simulink model "GyroSimulationAndIdentification_2016a"  (R2016a)
settings: Solver=ode45  SolverMode=SingleTasking  StartTime=0.0  StopTime=70.0  RelTol=1e-3
InitFcn:
  | InitGyro
values from neighbouring files (symbols this model uses):
  alpha1 = history1.x((2*m*(iter1-1) + m + 1):(2*m*iter1))    [PlotDualVariables.m]
  alpha1_star = history1.x((2*m*(iter1-1) + 1):(2*m*(iter1-1) + m))    [PlotDualVariables.m]
  alpha2 = history2.x((2*m*(iter2-1) + m + 1):(2*m*iter2))    [PlotDualVariables.m]
  alpha2_star = history2.x((2*m*(iter2-1) + 1):(2*m*(iter2-1) + m))    [PlotDualVariables.m]
  alpha3 = history3.x((2*m*(iter3-1) + m + 1):(2*m*iter3))    [PlotDualVariables.m]
  alpha3_star = history3.x((2*m*(iter3-1) + 1):(2*m*(iter3-1) + m))    [PlotDualVariables.m]
  alpha4 = history4.x((2*m*(iter4-1) + m + 1):(2*m*iter4))    [PlotDualVariables.m]
  alpha4_star = history4.x((2*m*(iter4-1) + 1):(2*m*(iter4-1) + m))    [PlotDualVariables.m]
  alpha5 = history5.x((2*m*(iter5-1) + m + 1):(2*m*iter5))    [PlotDualVariables.m]
  alpha5_star = history5.x((2*m*(iter5-1) + 1):(2*m*(iter5-1) + m))    [PlotDualVariables.m]
  alpha6 = history6.x((2*m*(iter6-1) + m + 1):(2*m*iter6))    [PlotDualVariables.m]
  alpha6_star = history6.x((2*m*(iter6-1) + 1):(2*m*(iter6-1) + m))    [PlotDualVariables.m]
  alpha7 = history7.x((2*m*(iter7-1) + m + 1):(2*m*iter7))    [PlotDualVariables.m]
  alpha7_star = history7.x((2*m*(iter7-1) + 1):(2*m*(iter7-1) + m))    [PlotDualVariables.m]
  alpha8 = history8.x((2*m*(iter8-1) + m + 1):(2*m*iter8))    [PlotDualVariables.m]
  alpha8_star = history8.x((2*m*(iter8-1) + 1):(2*m*(iter8-1) + m))    [PlotDualVariables.m]
  I_test = (1/m)*ones(1,m)    [Main.m]
  Im = (1/m)*ones(m,m)    [Main.m]
  K = zeros(m,m)    [Main.m]
  K_test = zeros(1,m)    [Main.m]
  Kernel_Var = 0.01    [Main.m]
  m = 100    [Main.m]
  n = 10    [Main.m]
  q1dot_0 = 45    [RunMe.m]
  q2_0 = 0    [RunMe.m]
  q3_0 = 0    [RunMe.m]
  rhodata = rho_data.data(1:5000,:)    [Main.m]
  xopt = [ydata(1:m,:) udata(1:m,:)]    [Main.m]
undefined symbols (not defined in the file or in its folder): Dr, Du, sigbuilder_block
undefined symbols (not defined in the file): sys
libraries: simulink_extras x5, simulink x2, cstblocks x1
settings Model: Creator=jt  LastModifiedBy=Saeed
settings DataIOCC: LimitDataPoints=on  SaveFormat=Array
settings OptimizationCC: BlockReduction=off  BooleanDataType=off
settings DebuggingCC: SaveWithParameterizedLinksMsg=none  UnderspecifiedInitializationDetection=Classic  MergeDetectMultiDrivingBlocksExec=none  SignalResolutionControl=TryResolveAllWithWarning
settings HardwareCC: ProdBitPerPointer=32  ProdLargestAtomicFloat=None  ProdIntDivRoundTo=Undefined  ProdEndianess=Unspecified  ProdWordSize=32  ProdHWDeviceType=32-bit Generic  TargetUnknown=on
settings ModelReferenceCC: PropagateSignalLabelsOutOfModel=off
settings ConfigComp: CovSFcnEnable=off

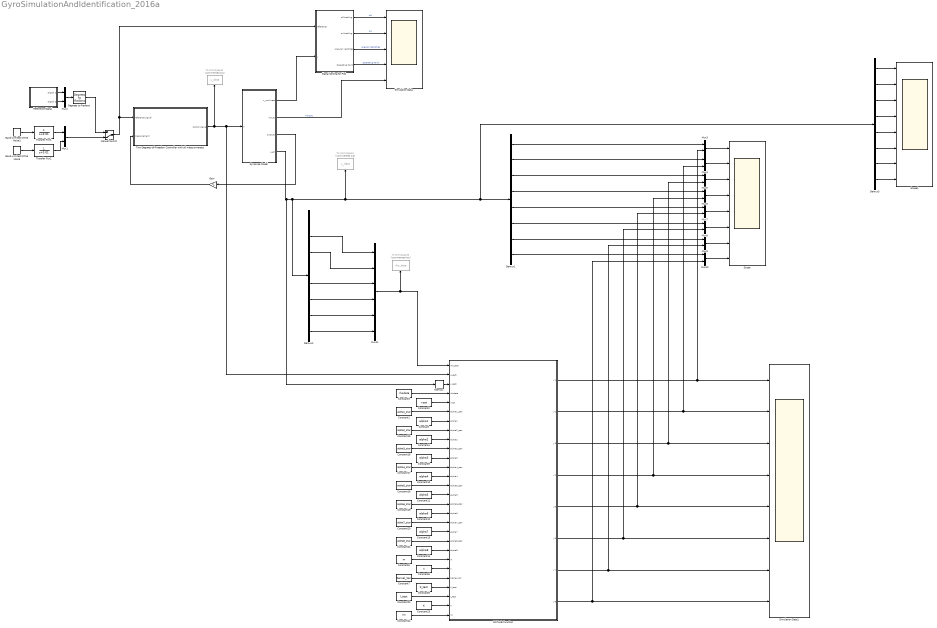
== system GyroSimulationAndIdentification_2016a ==
  Band-Limited White Noise : simulink/Sources/Band-Limited White Noise  Cov=[0.01]  Ts=0.01  seed=[3453]
  Band-Limited White Noise1 : simulink/Sources/Band-Limited White Noise  Cov=[0.01]  Ts=0.01  seed=[23341]
  Constant : Constant  Value=alpha1
  Constant1 : Constant  Value=alpha1_star
  Constant10 : Constant  Value=alpha4
  Constant11 : Constant  Value=alpha5
  Constant12 : Constant  Value=alpha6
  Constant13 : Constant  Value=alpha7
  Constant14 : Constant  Value=alpha8
  Constant15 : Constant  Value=alpha2_star
  Constant16 : Constant  Value=alpha3_star
  Constant17 : Constant  Value=alpha4_star
  Constant18 : Constant  Value=alpha5_star
  Constant19 : Constant  Value=alpha6_star
  Constant2 : Constant  Value=xopt
  Constant20 : Constant  Value=alpha7_star
  Constant21 : Constant  Value=alpha8_star
  Constant22 : Constant  Value=I_test
  Constant23 : Constant  Value=K
  Constant24 : Constant  Value=Im
  Constant3 : Constant  Value=rhodata
  Constant4 : Constant  Value=alpha2
  Constant5 : Constant  Value=m
  Constant6 : Constant  Value=n
  Constant7 : Constant  Value=Kernel_Var
  Constant8 : Constant  Value=K_test
  Constant9 : Constant  Value=alpha3
  Degrees to Radians : simulink_extras/Transformations/Degrees to Radians
  Demux1 : Demux  Outputs=8
  Demux2 : Demux  Outputs=8
  Demux3 : Demux  Outputs=8
  Gain : Gain  Gain=-1
  Gyroscpe Model : Subsystem
  MATLAB Function : MATLAB Function  TreatAsAtomicUnit=on
  Manual Switch : ManualSwitch  CurrentSetting=0
  Memory : Memory  X0=[0 q2_0 q3_0 0 q1dot_0 0 0 0];  InheritSampleTime=on  StateIdentifier=y_test
  Mux{1..10} (10 alike) : Mux  Inputs=2
  Mux11 : Mux  Inputs=6
  Reference Signal : Subsystem  Tag=STV Subsys  LoadFcn=sigbuilder_block('load');  StartFcn=sigbuilder_block('start');  StopFcn=sigbuilder_block('stop');  ClipboardFcn=sigbuilder_block('clipboard');  mask(Sigbuilder block){}
      mask help: Sigbuilder GUI
      mask init:
      | if ~strcmp(get_param(bdroot(gcbh),'SimulationStatus'),'stopped') tuvar = sigbuilder_block('maskInit'); end
      settings: CopyFcn=sigbuilder_block('copy');  DeleteFcn=sigbuilder_block('delete');  ModelCloseFcn=sigbuilder_block('modelClose');  PreSaveFcn=sigbuilder_block('preSave');  PauseFcn=sigbuilder_block('pause')  ContinueFcn=sigbuilder_block('continue')  NameChangeFcn=sigbuilder_block('namechange');  OpenFcn=sigbuilder_block('open',[6 0 1428 718.5 ]);  CloseFcn=sigbuilder_block('close');
      mask Display: plot(0, 0, 100, 100,[2, 2, 32, 32, 2], [68, 8, 8, 68, 68],[32, 2], [38, 38], [32, 19, 2],[53, 60, 44], [32, 17, 17, 2],[16, 16, 31, 31]);txt = getActiveGroup(gcbh);text(2, 100, txt,'verticalAlignment', 'top');
  Scope : Scope  NumInputPorts=8
  Scope1 : Scope  NumInputPorts=8
  Signal Sorting for Plot : Subsystem
  Simulation Data : Scope  NumInputPorts=5
  Simulation Data1 : Scope  NumInputPorts=8
  To Workspace1 : ToWorkspace  Commented=on  VariableName=y_data  SaveFormat=Timeseries  SampleTime=-1
  To Workspace2 : ToWorkspace  Commented=on  VariableName=u_data  SaveFormat=Timeseries  SampleTime=-1
  To Workspace3 : ToWorkspace  Commented=on  VariableName=rho_data  SaveFormat=Timeseries  SampleTime=-1
  Transfer Fcn1 : TransferFcn  Denominator=[1 0.01]
  Transfer Fcn2 : TransferFcn  Denominator=[1 0.01]
  Two-Degrees-of-Freedom Controller with all measurmenets : Subsystem
  wires:
  Gyroscpe Model/2(inputs) -> Simulation Data/5  "Torque"
  Gyroscpe Model/1(x_nonlinear) -> Signal Sorting for Plot/2(x)
  Mux2/1 -> Degrees to Radians/1
  Reference Signal/1(Signal 1) -> Mux2/1
  Reference Signal/2(Signal 2) -> Mux2/2
  Manual Switch/1 -> Signal Sorting for Plot/1(reference), Two-Degrees-of-Freedom Controller with all measurmenets/1(reference signal)
  Gyroscpe Model/3(outputs) -> Gain/1
  Signal Sorting for Plot/1(q3 tracking) -> Simulation Data/1  "q3"
  Signal Sorting for Plot/2(q4 tracking) -> Simulation Data/2  "q4"
  Signal Sorting for Plot/3(Angular velocities) -> Simulation Data/3  "Angular Velocities"
  Signal Sorting for Plot/4(Operating Point) -> Simulation Data/4  "Operating Point"
  Gain/1 -> Two-Degrees-of-Freedom Controller with all measurmenets/2(measurement)
  Two-Degrees-of-Freedom Controller with all measurmenets/1(control signal) -> MATLAB Function/2(u_test), Gyroscpe Model/1(T), To Workspace2/1
  Band-Limited White Noise1/1 -> Transfer Fcn1/1
  Band-Limited White Noise/1 -> Transfer Fcn2/1
  Degrees to Radians/1 -> Manual Switch/1
  Mux1/1 -> Manual Switch/2
  Transfer Fcn1/1 -> Mux1/1
  Transfer Fcn2/1 -> Mux1/2
  Gyroscpe Model/4(x_all) -> Memory/1, Demux2/1, Demux3/1, Demux1/1, To Workspace1/1
  Mux3/1 -> Scope/1
  Mux4/1 -> Scope/2
  Mux5/1 -> Scope/3
  Mux7/1 -> Scope/5
  Mux8/1 -> Scope/6
  Mux9/1 -> Scope/7
  Mux10/1 -> Scope/8
  Constant3/1 -> MATLAB Function/4(rhodata)
  Constant2/1 -> MATLAB Function/5(xopt)
  Constant1/1 -> MATLAB Function/6(alpha1_star)
  Constant/1 -> MATLAB Function/7(alpha1)
  Constant5/1 -> MATLAB Function/22(m)
  Constant6/1 -> MATLAB Function/23(n)
  Constant8/1 -> MATLAB Function/25(K_test)
  Constant7/1 -> MATLAB Function/24(Kernel_Var)
  Constant4/1 -> MATLAB Function/9(alpha2)
  Constant9/1 -> MATLAB Function/11(alpha3)
  Constant10/1 -> MATLAB Function/13(alpha4)
  Constant11/1 -> MATLAB Function/15(alpha5)
  Constant12/1 -> MATLAB Function/17(alpha6)
  Constant13/1 -> MATLAB Function/19(alpha7)
  Constant14/1 -> MATLAB Function/21(alpha8)
  Constant15/1 -> MATLAB Function/8(alpha2_star)
  Constant16/1 -> MATLAB Function/10(alpha3_star)
  Constant17/1 -> MATLAB Function/12(alpha4_star)
  Constant18/1 -> MATLAB Function/14(alpha5_star)
  Constant19/1 -> MATLAB Function/16(alpha6_star)
  Constant20/1 -> MATLAB Function/18(alpha7_star)
  Constant21/1 -> MATLAB Function/20(alpha8_star)
  Memory/1 -> MATLAB Function/3(y_test)
  MATLAB Function/1(y1) -> Mux3/2, Simulation Data1/1
  MATLAB Function/2(y2) -> Mux4/2, Simulation Data1/2
  MATLAB Function/3(y3) -> Mux5/2, Simulation Data1/3
  MATLAB Function/4(y4) -> Mux6/2, Simulation Data1/4
  MATLAB Function/5(y5) -> Mux7/2, Simulation Data1/5
  MATLAB Function/6(y6) -> Mux8/2, Simulation Data1/6
  MATLAB Function/7(y7) -> Mux9/2, Simulation Data1/7
  MATLAB Function/8(y8) -> Mux10/2, Simulation Data1/8
  Demux1/1 -> Mux3/1
  Demux1/2 -> Mux4/1
  Demux1/3 -> Mux5/1
  Demux1/4 -> Mux6/1
  Demux1/5 -> Mux7/1
  Demux1/6 -> Mux8/1
  Demux1/7 -> Mux9/1
  Demux1/8 -> Mux10/1
  Mux11/1 -> To Workspace3/1, MATLAB Function/1(rho_test)
  Mux6/1 -> Scope/4
  Demux2/2 -> Mux11/1
  Demux2/3 -> Mux11/2
  Demux2/5 -> Mux11/3
  Demux2/6 -> Mux11/4
  Demux2/8 -> Mux11/6
  Demux2/7 -> Mux11/5
  Demux3/1 -> Scope1/1
  Demux3/2 -> Scope1/2
  Demux3/3 -> Scope1/3
  Demux3/4 -> Scope1/4
  Demux3/5 -> Scope1/5
  Demux3/6 -> Scope1/6
  Demux3/8 -> Scope1/8
  Demux3/7 -> Scope1/7
  Constant22/1 -> MATLAB Function/26(I_test)
  Constant23/1 -> MATLAB Function/27(K)
  Constant24/1 -> MATLAB Function/28(Im)

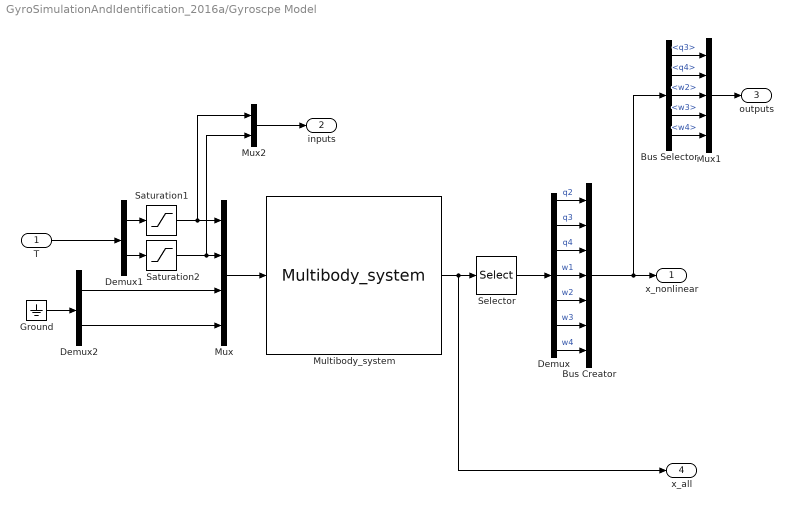
== system GyroSimulationAndIdentification_2016a/Gyroscpe Model ==
  T : Inport
  Bus Creator : BusCreator  Inputs=7
  Bus Selector : BusSelector  OutputSignals=q3,q4,w2,w3,w4
  Demux : Demux  Outputs=7
  Demux1 : Demux  Outputs=2
  Demux2 : Demux  Outputs=2
  Ground : Ground
  Multibody_system : S-Function  FunctionName=Multibody_system  Parameters=paraStruct, initY, initDy  SFunctionDeploymentMode=off  EnableBusSupport=off  mask(Neweul-M2 nonlinear model){paraStruct=sys.parameters.data, initY=[0 q2_0 q3_0 0]';, initDy=[q1dot_0 0 0 0]';}
      mask prompts: paraStruct "Neweul-M2 Parameter Structure"; initY "Initial coordinates"; initDy "Initial velocities"
      mask help:
      | State-state representation of a multibody system
      | created with Neueul-MÂ².
      |
      | In order to run a simulation in Simulink you have to provide
      | the following input parameters:
      |   * Neweul-M2 Parameter Structure (sys.parameters.data)
      |     ... Structure containing all user-defined parameters
      |   * Initial coordinates (zeros(sys.counters.genCoord,1))
      |     ... Initial values for the generalized coordinates
      |   * Initial velocities (zeros(sys.dof,1))
      |     ... Initial values for the generalized velocities
      |
      | Neweul-MÂ²
      | Multibody systems based on symbolic Newton-Euler-Equations
      | Copyright (c) ITM University of Stuttgart, www.itm.uni-stuttgart.de
      mask Display:
      | port_label('output',1,'states [8x1]');
      | port_label('input',1,'control [4x1]');
  Mux : Mux
  Mux1 : Mux  Inputs=5
  Mux2 : Mux  Inputs=2
  Saturation1 : Saturate  UpperLimit=0.666  LowerLimit=-0.666
  Saturation2 : Saturate  UpperLimit=2.44  LowerLimit=-2.44
  Selector : Selector  IndexOptions=Index vector (dialog)  Indices=2:8  OutputSizes=1
  x_nonlinear : Outport
  inputs : Outport  Port=2
  outputs : Outport  Port=3
  x_all : Outport  Port=4
  wires:
  Multibody_system/1 -> x_all/1, Selector/1
  Demux/6 -> Bus Creator/6  "w3"
  Demux/3 -> Bus Creator/3  "q4"
  Demux/1 -> Bus Creator/1  "q2"
  Demux/2 -> Bus Creator/2  "q3"
  Demux/7 -> Bus Creator/7  "w4"
  Selector/1 -> Demux/1
  Bus Creator/1 -> Bus Selector/1, x_nonlinear/1
  Mux/1 -> Multibody_system/1
  Demux2/2 -> Mux/4
  Demux2/1 -> Mux/3
  Demux1/2 -> Saturation2/1
  Demux/5 -> Bus Creator/5  "w2"
  Demux/4 -> Bus Creator/4  "w1"
  Mux2/1 -> inputs/1
  Saturation2/1 -> Mux2/2, Mux/2
  Saturation1/1 -> Mux2/1, Mux/1
  Mux1/1 -> outputs/1
  Demux1/1 -> Saturation1/1
  T/1 -> Demux1/1
  Ground/1 -> Demux2/1
  Bus Selector/1 -> Mux1/1  "<q3>"
  Bus Selector/2 -> Mux1/2  "<q4>"
  Bus Selector/3 -> Mux1/3  "<w2>"
  Bus Selector/4 -> Mux1/4  "<w3>"
  Bus Selector/5 -> Mux1/5  "<w4>"

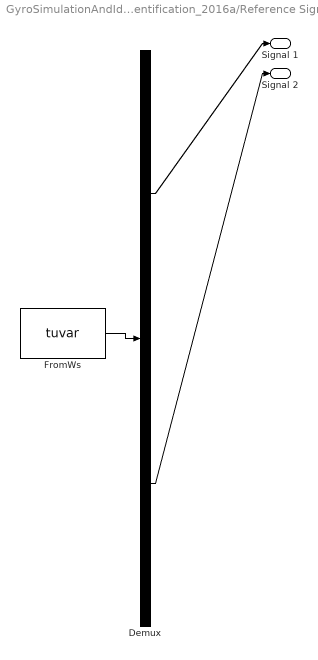
== system GyroSimulationAndIdentification_2016a/Reference Signal ==
  Demux : Demux  Tag=STV Demux  Outputs=2
  FromWs : FromWorkspace  Tag=STV FromWs  VariableName=tuvar  SampleTime=0
      SigBuilderData=|
      | common.afterFinalStr = 'Extrapolate'
      | common.sampleTime = 0
      | dataSet.timeRange = [0 70]
      | dataSet.name = 'Group 1'
      | sbobj.Groups.Name = 'Group 1'
      | sbobj.Groups.Signals(1).Name = 'Signal 1'
      | sbobj.Groups.Signals(1).XData = [0 22 22 28 28 34 34 40 40 46 46 52 52 58 58 64 64 70]
      | sbobj.Groups.Signals(1).YData = [0 0 -5 -5 0 0 5 5 0 0 -5 -5 0 0 5 5 0 0]
      | sbobj.Groups.Signals(2).Name = 'Signal 2'
      | sbobj.Groups.Signals(2).XData = [0 25 25 37 37 49 49 61 61 70]
      | sbobj.Groups.Signals(2).YData = [0 0 -40 -40 0 -0.2 40 40 -0.2 -0.2]
      | sbobj.Groups.TimeRange = [0 70]
  Signal 1 : Outport  Tag=STV Outport
  Signal 2 : Outport  Tag=STV Outport  Port=2
  wires:
  FromWs/1 -> Demux/1
  Demux/1 -> Signal 1/1
  Demux/2 -> Signal 2/1

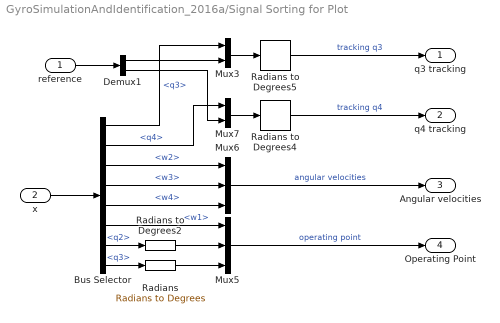
== system GyroSimulationAndIdentification_2016a/Signal Sorting for Plot ==
  reference : Inport
  x : Inport  Port=2
  Bus Selector : BusSelector  OutputSignals=q3,q4,w2,w3,w4,w1,q2,q3
  Demux1 : Demux  Outputs=2
  Mux3 : Mux  Inputs=2
  Mux5 : Mux  Inputs=3
  Mux6 : Mux  Inputs=3
  Mux7 : Mux  Inputs=2
  "Radians " : simulink_extras/Transformations/Radians to Degrees
  Radians to Degrees2 : simulink_extras/Transformations/Radians to Degrees
  Radians to Degrees4 : simulink_extras/Transformations/Radians to Degrees
  Radians to Degrees5 : simulink_extras/Transformations/Radians to Degrees
  q3 tracking : Outport
  q4 tracking : Outport  Port=2
  Angular velocities : Outport  Port=3
  Operating Point : Outport  Port=4
  wires:
  Bus Selector/3 -> Mux6/1  "<w2>"
  Bus Selector/2 -> Mux7/1  "<q4>"
  Radians to Degrees4/1 -> q4 tracking/1  "tracking q4"
  Mux3/1 -> Radians to Degrees5/1
  Radians to Degrees5/1 -> q3 tracking/1  "tracking q3"
  Mux7/1 -> Radians to Degrees4/1
  Demux1/1 -> Mux3/2
  Demux1/2 -> Mux7/2
  Bus Selector/1 -> Mux3/1  "<q3>"
  Mux6/1 -> Angular velocities/1  "angular velocities"
  Bus Selector/5 -> Mux6/3  "<w4>"
  Bus Selector/4 -> Mux6/2  "<w3>"
  Mux5/1 -> Operating Point/1  "operating point"
  Bus Selector/6 -> Mux5/1  "<w1>"
  Bus Selector/7 -> Radians to Degrees2/1  "<q2>"
  Bus Selector/8 -> "Radians "/1  "<q3>"
  "Radians "/1 -> Mux5/3
  Radians to Degrees2/1 -> Mux5/2
  reference/1 -> Demux1/1
  x/1 -> Bus Selector/1

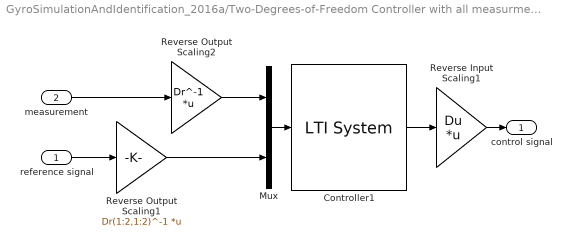
== system GyroSimulationAndIdentification_2016a/Two-Degrees-of-Freedom Controller with all measurmenets ==
  reference signal : Inport
  measurement : Inport  Port=2
  Controller1 : cstblocks/LTI System  sys=K3  IC=[]
  Mux : Mux  Inputs=2
  Reverse Input Scaling1 : Gain  Gain=Du  Multiplication=Matrix(K*u)
  Reverse Output Scaling1 : Gain  Gain=Dr(1:2,1:2)^-1  Multiplication=Matrix(K*u)
  Reverse Output Scaling2 : Gain  Gain=Dr^-1  Multiplication=Matrix(K*u)
  control signal : Outport
  wires:
  Reverse Output Scaling1/1 -> Mux/2
  Reverse Output Scaling2/1 -> Mux/1
  measurement/1 -> Reverse Output Scaling2/1
  Mux/1 -> Controller1/1
  Controller1/1 -> Reverse Input Scaling1/1
  Reverse Input Scaling1/1 -> control signal/1
  reference signal/1 -> Reverse Output Scaling1/1

== matlab function GyroSimulationAndIdentification_2016a/MATLAB Function ==
  data: rho_test input size=[1,6]; y1 output size=1; u_test input size=[1,2]; y_test input size=[1,8]; rhodata input size=[5000,6]; xopt input size=[100,10]; alpha1_star input size=[100,1]; alpha1 input size=[100,1]; alpha2_star input size=[100,1]; alpha2 input size=[100,1]; alpha3_star input size=[100,1]; alpha3 input size=[100,1]; alpha4_star input size=[100,1]; alpha4 input size=[100,1]; alpha5_star input size=[100,1]; alpha5 input size=[100,1]; alpha6_star input size=[100,1]; alpha6 input size=[100,1]; alpha7_star input size=[100,1]; alpha7 input size=[100,1]; alpha8_star input size=[100,1]; alpha8 input size=[100,1]; m input size=1; n input size=1; Kernel_Var input size=1; K_test input size=[1,100]; y2 output size=1; y3 output size=1; y4 output size=1; y5 output size=1; y6 output size=1; y7 output size=1; y8 output size=1; I_test input size=[1,100]; K input size=[100,100]; Im input size=[100,100]
function [y1 ,y2 ,y3 ,y4 ,y5 ,y6 ,y7 ,y8]= fcn(rho_test, u_test, y_test, rhodata, xopt, alpha1_star, alpha1, alpha2_star, alpha2, alpha3_star, alpha3, alpha4_star, alpha4, alpha5_star, alpha5, alpha6_star, alpha6, alpha7_star, alpha7, alpha8_star, alpha8, m, n, Kernel_Var, K_test, I_test, K, Im)


u_test = [u_test(1) u_test(2)];
y_test = [y_test(1) y_test(2) y_test(3) y_test(4) y_test(5) y_test(6) y_test(7) y_test(8)];
x_test = [y_test u_test];


%% Constructs the test Kernel Matrix and Center the points 
for i = 1:m
    xright = xopt(i,:);
    for k = 1:n
    K_test(1,i) = K_test(1,i) + x_test(k)*exp(-(norm(rho_test-rhodata(i,:))^2)/Kernel_Var)*xright(k);
    end
end
K_test_Centered = K_test - (I_test*K) - (K_test*Im) + (I_test*K*Im);

%% Computes the test points, Computes each component of a test point with respect tp its corresponding dual variables coming from the optimization problem 

y1 = K_test_Centered*(alpha1_star - alpha1);
y2 = K_test_Centered*(alpha2_star - alpha2);
y3 = K_test_Centered*(alpha3_star - alpha3);
y4 = K_test_Centered*(alpha4_star - alpha4);
y5 = K_test_Centered*(alpha5_star - alpha5);
y6 = K_test_Centered*(alpha6_star - alpha6);
y7 = K_test_Centered*(alpha7_star - alpha7);
y8 = K_test_Centered*(alpha8_star - alpha8);
